simulink model "db5_6_Level_double"  (R2021a)
settings: Solver=VariableStepAuto  StartTime=0.0  StopTime=8  RelTol=1e-3
undefined symbols (not defined in the file): lambda2
libraries: dspsigops x13, dspquant2 x1
(part 2 of 4)

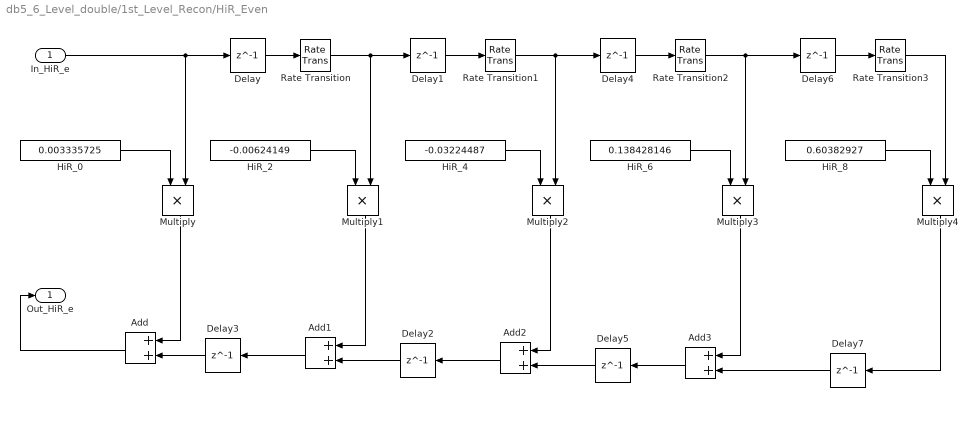
== system db5_6_Level_double/1st_Level_Recon/HiR_Even ==
  In_HiR_e : Inport  OutDataTypeStr=double  SampleTime=1/44100
  Add{,1..3} (4 alike) : Sum  AccumDataTypeStr=double  OutDataTypeStr=double
  Delay{,1..7} (8 alike) : Delay  DelayLength=1  SampleTime=1/44100
  HiR_0 : Constant  Value=0.003335725  OutDataTypeStr=double  SampleTime=1/44100
  HiR_2 : Constant  Value=-0.00624149  OutDataTypeStr=double  SampleTime=1/44100
  HiR_4 : Constant  Value=-0.03224487  OutDataTypeStr=double  SampleTime=1/44100
  HiR_6 : Constant  Value=0.138428146  OutDataTypeStr=double  SampleTime=1/44100
  HiR_8 : Constant  Value=0.60382927  OutDataTypeStr=double  SampleTime=1/44100
  Multiply{,1..4} (5 alike) : Product  OutDataTypeStr=double
  Rate Transition{,1..3} (4 alike) : RateTransition  OutPortSampleTime=1/44100
  Out_HiR_e : Outport  OutDataTypeStr=double  SampleTime=1/44100  VectorParamsAs1DForOutWhenUnconnected=off
  wires:
  Delay3/1 -> Add/2
  In_HiR_e/1 -> Delay/1, Multiply/2
  HiR_4/1 -> Multiply2/1
  Multiply/1 -> Add/1
  Add1/1 -> Delay3/1
  Multiply1/1 -> Add1/1
  Delay2/1 -> Add1/2
  Add/1 -> Out_HiR_e/1
  HiR_0/1 -> Multiply/1
  HiR_2/1 -> Multiply1/1
  Delay1/1 -> Rate Transition1/1
  Rate Transition/1 -> Delay1/1, Multiply1/2
  Rate Transition1/1 -> Delay4/1, Multiply2/2
  Delay/1 -> Rate Transition/1
  Delay4/1 -> Rate Transition2/1
  HiR_6/1 -> Multiply3/1
  Multiply2/1 -> Add2/1
  Add2/1 -> Delay2/1
  Delay5/1 -> Add2/2
  Rate Transition3/1 -> Multiply4/2
  Multiply4/1 -> Delay7/1
  HiR_8/1 -> Multiply4/1
  Rate Transition2/1 -> Delay6/1, Multiply3/2
  Delay6/1 -> Rate Transition3/1
  Add3/1 -> Delay5/1
  Multiply3/1 -> Add3/1
  Delay7/1 -> Add3/2

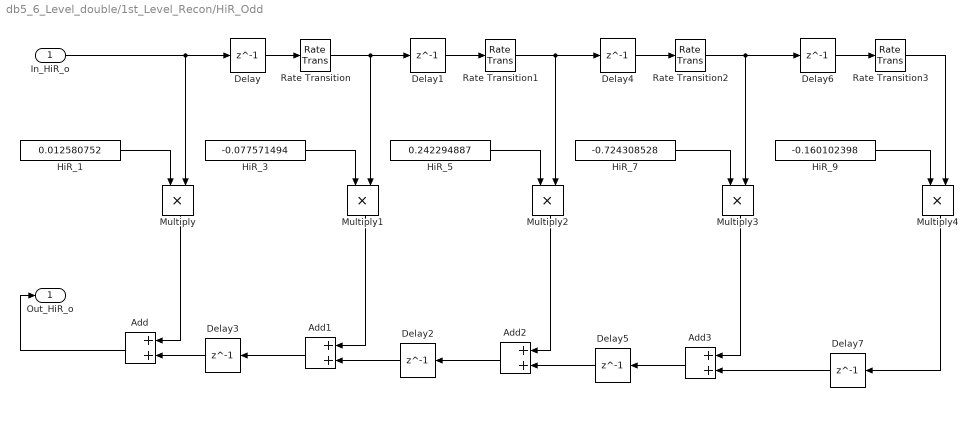
== system db5_6_Level_double/1st_Level_Recon/HiR_Odd ==
  In_HiR_o : Inport  OutDataTypeStr=double  SampleTime=1/44100
  Add{,1..3} (4 alike) : Sum  AccumDataTypeStr=double  OutDataTypeStr=double
  Delay{,1..7} (8 alike) : Delay  DelayLength=1  SampleTime=1/44100
  HiR_1 : Constant  Value=0.012580752  OutDataTypeStr=double  SampleTime=1/44100
  HiR_3 : Constant  Value=-0.077571494  OutDataTypeStr=double  SampleTime=1/44100
  HiR_5 : Constant  Value=0.242294887  OutDataTypeStr=double  SampleTime=1/44100
  HiR_7 : Constant  Value=-0.724308528  OutDataTypeStr=double  SampleTime=1/44100
  HiR_9 : Constant  Value=-0.160102398  OutDataTypeStr=double  SampleTime=1/44100
  Multiply{,1..4} (5 alike) : Product  OutDataTypeStr=double
  Rate Transition{,1..3} (4 alike) : RateTransition  OutPortSampleTime=1/44100
  Out_HiR_o : Outport  OutDataTypeStr=double  SampleTime=1/44100  VectorParamsAs1DForOutWhenUnconnected=off
  wires:
  Add/1 -> Out_HiR_o/1
  Add2/1 -> Delay2/1
  Delay5/1 -> Add2/2
  HiR_9/1 -> Multiply4/1
  HiR_5/1 -> Multiply2/1
  HiR_1/1 -> Multiply/1
  HiR_7/1 -> Multiply3/1
  Multiply1/1 -> Add1/1
  Multiply2/1 -> Add2/1
  Delay2/1 -> Add1/2
  Delay4/1 -> Rate Transition2/1
  Delay3/1 -> Add/2
  In_HiR_o/1 -> Delay/1, Multiply/2
  Rate Transition/1 -> Delay1/1, Multiply1/2
  Rate Transition2/1 -> Delay6/1, Multiply3/2
  Delay7/1 -> Add3/2
  Delay6/1 -> Rate Transition3/1
  Add3/1 -> Delay5/1
  Rate Transition3/1 -> Multiply4/2
  HiR_3/1 -> Multiply1/1
  Multiply3/1 -> Add3/1
  Add1/1 -> Delay3/1
  Multiply4/1 -> Delay7/1
  Multiply/1 -> Add/1
  Rate Transition1/1 -> Delay4/1, Multiply2/2
  Delay1/1 -> Rate Transition1/1
  Delay/1 -> Rate Transition/1

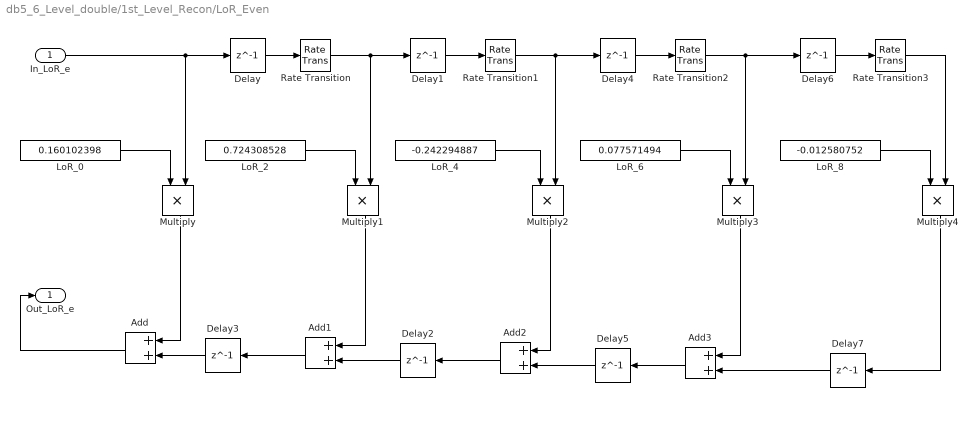
== system db5_6_Level_double/1st_Level_Recon/LoR_Even ==
  In_LoR_e : Inport  OutDataTypeStr=double  SampleTime=1/44100
  Add{,1..3} (4 alike) : Sum  AccumDataTypeStr=double  OutDataTypeStr=double
  Delay{,1..7} (8 alike) : Delay  DelayLength=1  SampleTime=1/44100
  LoR_0 : Constant  Value=0.160102398  OutDataTypeStr=double  SampleTime=1/44100
  LoR_2 : Constant  Value=0.724308528  OutDataTypeStr=double  SampleTime=1/44100
  LoR_4 : Constant  Value=-0.242294887  OutDataTypeStr=double  SampleTime=1/44100
  LoR_6 : Constant  Value=0.077571494  OutDataTypeStr=double  SampleTime=1/44100
  LoR_8 : Constant  Value=-0.012580752  OutDataTypeStr=double  SampleTime=1/44100
  Multiply{,1..4} (5 alike) : Product  OutDataTypeStr=double
  Rate Transition{,1..3} (4 alike) : RateTransition  OutPortSampleTime=1/44100
  Out_LoR_e : Outport  OutDataTypeStr=double  SampleTime=1/44100  VectorParamsAs1DForOutWhenUnconnected=off
  wires:
  Add2/1 -> Delay2/1
  Delay5/1 -> Add2/2
  Add/1 -> Out_LoR_e/1
  Delay1/1 -> Rate Transition1/1
  Rate Transition1/1 -> Delay4/1, Multiply2/2
  Multiply/1 -> Add/1
  Add1/1 -> Delay3/1
  Delay/1 -> Rate Transition/1
  Multiply2/1 -> Add2/1
  Multiply1/1 -> Add1/1
  Delay3/1 -> Add/2
  Delay4/1 -> Rate Transition2/1
  Delay2/1 -> Add1/2
  Rate Transition/1 -> Delay1/1, Multiply1/2
  In_LoR_e/1 -> Delay/1, Multiply/2
  LoR_4/1 -> Multiply2/1
  Delay6/1 -> Rate Transition3/1
  LoR_0/1 -> Multiply/1
  Delay7/1 -> Add3/2
  Rate Transition2/1 -> Delay6/1, Multiply3/2
  LoR_8/1 -> Multiply4/1
  LoR_2/1 -> Multiply1/1
  Rate Transition3/1 -> Multiply4/2
  LoR_6/1 -> Multiply3/1
  Multiply4/1 -> Delay7/1
  Multiply3/1 -> Add3/1
  Add3/1 -> Delay5/1

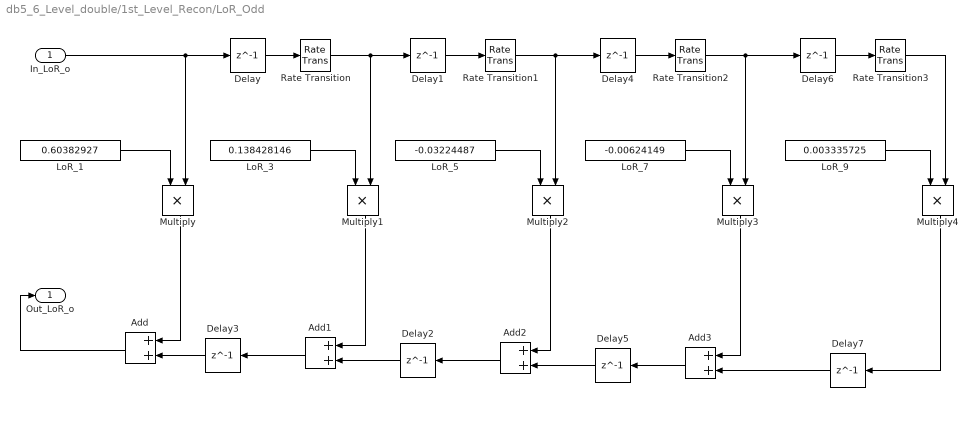
== system db5_6_Level_double/1st_Level_Recon/LoR_Odd ==
  In_LoR_o : Inport  OutDataTypeStr=double  SampleTime=1/44100
  Add{,1..3} (4 alike) : Sum  AccumDataTypeStr=double  OutDataTypeStr=double
  Delay{,1..7} (8 alike) : Delay  DelayLength=1  SampleTime=1/44100
  LoR_1 : Constant  Value=0.60382927  OutDataTypeStr=double  SampleTime=1/44100
  LoR_3 : Constant  Value=0.138428146  OutDataTypeStr=double  SampleTime=1/44100
  LoR_5 : Constant  Value=-0.03224487  OutDataTypeStr=double  SampleTime=1/44100
  LoR_7 : Constant  Value=-0.00624149  OutDataTypeStr=double  SampleTime=1/44100
  LoR_9 : Constant  Value=0.003335725  OutDataTypeStr=double  SampleTime=1/44100
  Multiply{,1..4} (5 alike) : Product  OutDataTypeStr=double
  Rate Transition{,1..3} (4 alike) : RateTransition  OutPortSampleTime=1/44100
  Out_LoR_o : Outport  OutDataTypeStr=double  SampleTime=1/44100  VectorParamsAs1DForOutWhenUnconnected=off
  wires:
  LoR_9/1 -> Multiply4/1
  Rate Transition2/1 -> Delay6/1, Multiply3/2
  Rate Transition/1 -> Delay1/1, Multiply1/2
  Rate Transition3/1 -> Multiply4/2
  Add3/1 -> Delay5/1
  Delay6/1 -> Rate Transition3/1
  Delay7/1 -> Add3/2
  LoR_1/1 -> Multiply/1
  LoR_3/1 -> Multiply1/1
  Delay3/1 -> Add/2
  Delay4/1 -> Rate Transition2/1
  LoR_5/1 -> Multiply2/1
  Delay2/1 -> Add1/2
  Multiply2/1 -> Add2/1
  Add2/1 -> Delay2/1
  LoR_7/1 -> Multiply3/1
  Delay5/1 -> Add2/2
  Multiply3/1 -> Add3/1
  Multiply/1 -> Add/1
  Delay1/1 -> Rate Transition1/1
  Multiply4/1 -> Delay7/1
  In_LoR_o/1 -> Delay/1, Multiply/2
  Add1/1 -> Delay3/1
  Add/1 -> Out_LoR_o/1
  Rate Transition1/1 -> Delay4/1, Multiply2/2
  Delay/1 -> Rate Transition/1
  Multiply1/1 -> Add1/1

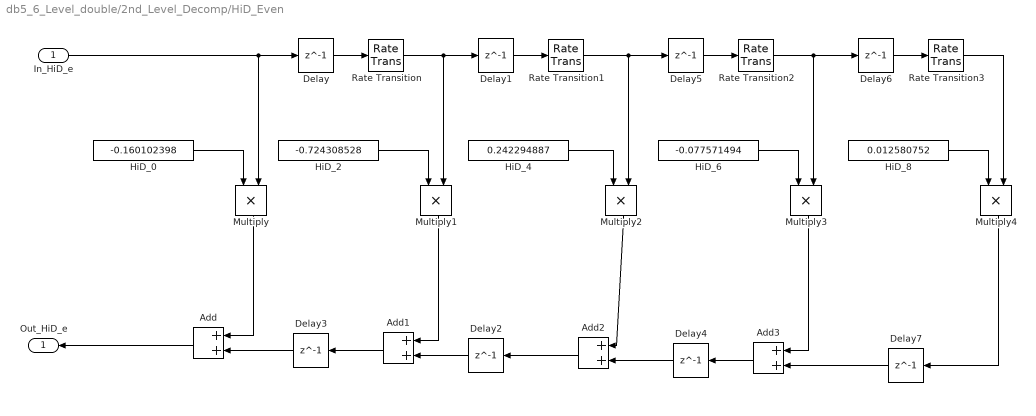
== system db5_6_Level_double/2nd_Level_Decomp/HiD_Even ==
  In_HiD_e : Inport  OutDataTypeStr=double  SampleTime=1/44100
  Add{,1..3} (4 alike) : Sum  AccumDataTypeStr=double  OutDataTypeStr=double
  Delay{,1..7} (8 alike) : Delay  DelayLength=1  SampleTime=1/44100
  HiD_0 : Constant  Value=-0.160102398  OutDataTypeStr=double  SampleTime=1/44100
  HiD_2 : Constant  Value=-0.724308528  OutDataTypeStr=double  SampleTime=1/44100
  HiD_4 : Constant  Value=0.242294887  OutDataTypeStr=double  SampleTime=1/44100
  HiD_6 : Constant  Value=-0.077571494  OutDataTypeStr=double  SampleTime=1/44100
  HiD_8 : Constant  Value=0.012580752  OutDataTypeStr=double  SampleTime=1/44100
  Multiply{,1..4} (5 alike) : Product  OutDataTypeStr=double
  Rate Transition{,1..3} (4 alike) : RateTransition  OutPortSampleTime=1/44100
  Out_HiD_e : Outport  OutDataTypeStr=double  SampleTime=1/44100  VectorParamsAs1DForOutWhenUnconnected=off
  wires:
  Delay1/1 -> Rate Transition1/1
  Delay3/1 -> Add/2
  HiD_2/1 -> Multiply1/1
  Rate Transition2/1 -> Delay6/1, Multiply3/2
  Add/1 -> Out_HiD_e/1
  Delay4/1 -> Add2/2
  Delay5/1 -> Rate Transition2/1
  Rate Transition1/1 -> Delay5/1, Multiply2/2
  HiD_0/1 -> Multiply/1
  Multiply2/1 -> Add2/1
  Add2/1 -> Delay2/1
  HiD_6/1 -> Multiply3/1
  Multiply/1 -> Add/1
  In_HiD_e/1 -> Delay/1, Multiply/2
  Multiply1/1 -> Add1/1
  Rate Transition/1 -> Delay1/1, Multiply1/2
  Add1/1 -> Delay3/1
  HiD_4/1 -> Multiply2/1
  Delay/1 -> Rate Transition/1
  Delay2/1 -> Add1/2
  HiD_8/1 -> Multiply4/1
  Delay6/1 -> Rate Transition3/1
  Rate Transition3/1 -> Multiply4/2
  Multiply4/1 -> Delay7/1
  Multiply3/1 -> Add3/1
  Add3/1 -> Delay4/1
  Delay7/1 -> Add3/2

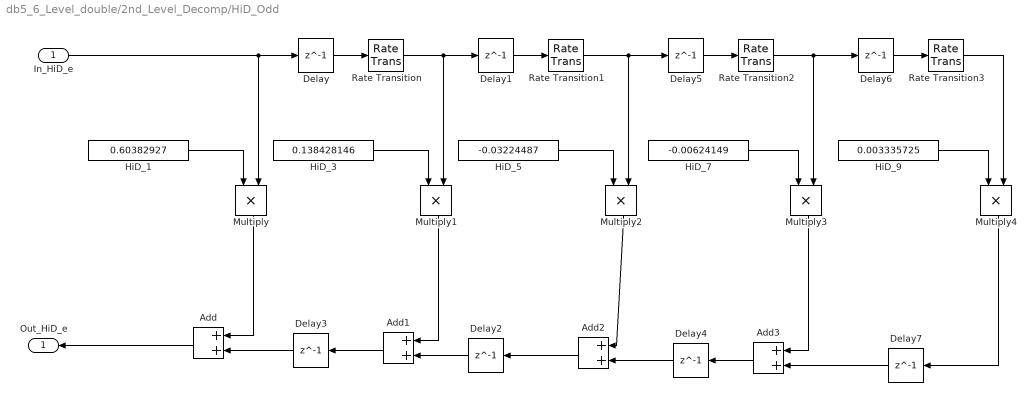
== system db5_6_Level_double/2nd_Level_Decomp/HiD_Odd ==
  In_HiD_e : Inport  OutDataTypeStr=double  SampleTime=1/44100
  Add{,1..3} (4 alike) : Sum  AccumDataTypeStr=double  OutDataTypeStr=double
  Delay{,1..7} (8 alike) : Delay  DelayLength=1  SampleTime=1/44100
  HiD_1 : Constant  Value=0.60382927  OutDataTypeStr=double  SampleTime=1/44100
  HiD_3 : Constant  Value=0.138428146  OutDataTypeStr=double  SampleTime=1/44100
  HiD_5 : Constant  Value=-0.03224487  OutDataTypeStr=double  SampleTime=1/44100
  HiD_7 : Constant  Value=-0.00624149  OutDataTypeStr=double  SampleTime=1/44100
  HiD_9 : Constant  Value=0.003335725  OutDataTypeStr=double  SampleTime=1/44100
  Multiply{,1..4} (5 alike) : Product  OutDataTypeStr=double
  Rate Transition{,1..3} (4 alike) : RateTransition  OutPortSampleTime=1/44100
  Out_HiD_e : Outport  OutDataTypeStr=double  SampleTime=1/44100  VectorParamsAs1DForOutWhenUnconnected=off
  wires:
  Multiply4/1 -> Delay7/1
  Delay6/1 -> Rate Transition3/1
  Rate Transition3/1 -> Multiply4/2
  Add3/1 -> Delay4/1
  Add/1 -> Out_HiD_e/1
  Delay1/1 -> Rate Transition1/1
  Delay7/1 -> Add3/2
  Rate Transition2/1 -> Delay6/1, Multiply3/2
  Delay3/1 -> Add/2
  Rate Transition/1 -> Delay1/1, Multiply1/2
  Rate Transition1/1 -> Delay5/1, Multiply2/2
  Delay4/1 -> Add2/2
  Multiply/1 -> Add/1
  Add2/1 -> Delay2/1
  Delay5/1 -> Rate Transition2/1
  Multiply1/1 -> Add1/1
  Delay2/1 -> Add1/2
  Delay/1 -> Rate Transition/1
  Add1/1 -> Delay3/1
  Multiply3/1 -> Add3/1
  HiD_3/1 -> Multiply1/1
  Multiply2/1 -> Add2/1
  HiD_7/1 -> Multiply3/1
  In_HiD_e/1 -> Delay/1, Multiply/2
  HiD_1/1 -> Multiply/1
  HiD_5/1 -> Multiply2/1
  HiD_9/1 -> Multiply4/1

== system db5_6_Level_double/2nd_Level_Decomp/LoD_Even ==
  In_HiD_e : Inport  OutDataTypeStr=double  SampleTime=1/44100
  Add{,1..3} (4 alike) : Sum  AccumDataTypeStr=double  OutDataTypeStr=double
  Delay{,1..7} (8 alike) : Delay  DelayLength=1  SampleTime=1/44100
  LoD_0 : Constant  Value=0.003335725  OutDataTypeStr=double  SampleTime=1/44100
  LoD_2 : Constant  Value=-0.00624149  OutDataTypeStr=double  SampleTime=1/44100
  LoD_4 : Constant  Value=-0.03224487  OutDataTypeStr=double  SampleTime=1/44100
  LoD_6 : Constant  Value=0.138428146  OutDataTypeStr=double  SampleTime=1/44100
  LoD_8 : Constant  Value=0.60382927  OutDataTypeStr=double  SampleTime=1/44100
  Multiply{,1..4} (5 alike) : Product  OutDataTypeStr=double
  Rate Transition{,1..3} (4 alike) : RateTransition  OutPortSampleTime=1/44100
  Out_HiD_e : Outport  OutDataTypeStr=double  SampleTime=1/44100  VectorParamsAs1DForOutWhenUnconnected=off
  wires:
  Multiply3/1 -> Add3/1
  LoD_4/1 -> Multiply2/1
  Multiply2/1 -> Add2/1
  Add1/1 -> Delay3/1
  Delay2/1 -> Add1/2
  Delay/1 -> Rate Transition/1
  Multiply1/1 -> Add1/1
  In_HiD_e/1 -> Delay/1, Multiply/2
  Add2/1 -> Delay2/1
  Delay5/1 -> Rate Transition2/1
  Multiply/1 -> Add/1
  LoD_8/1 -> Multiply4/1
  Delay4/1 -> Add2/2
  Rate Transition1/1 -> Delay5/1, Multiply2/2
  Rate Transition/1 -> Delay1/1, Multiply1/2
  Delay3/1 -> Add/2
  Rate Transition2/1 -> Delay6/1, Multiply3/2
  Add/1 -> Out_HiD_e/1
  Delay1/1 -> Rate Transition1/1
  Delay7/1 -> Add3/2
  LoD_6/1 -> Multiply3/1
  Add3/1 -> Delay4/1
  Rate Transition3/1 -> Multiply4/2
  Delay6/1 -> Rate Transition3/1
  Multiply4/1 -> Delay7/1
  LoD_2/1 -> Multiply1/1
  LoD_0/1 -> Multiply/1

== system db5_6_Level_double/2nd_Level_Decomp/LoD_Odd ==
  In_HiD_e : Inport  OutDataTypeStr=double  SampleTime=1/44100
  Add{,1..3} (4 alike) : Sum  AccumDataTypeStr=double  OutDataTypeStr=double
  Delay{,1..7} (8 alike) : Delay  DelayLength=1  SampleTime=1/44100
  LoD_1 : Constant  Value=-0.012580752  OutDataTypeStr=double  SampleTime=1/44100
  LoD_3 : Constant  Value=0.077571494  OutDataTypeStr=double  SampleTime=1/44100
  LoD_5 : Constant  Value=-0.242294887  OutDataTypeStr=double  SampleTime=1/44100
  LoD_7 : Constant  Value=0.724308528  OutDataTypeStr=double  SampleTime=1/44100
  LoD_9 : Constant  Value=0.160102398  OutDataTypeStr=double  SampleTime=1/44100
  Multiply{,1..4} (5 alike) : Product  OutDataTypeStr=double
  Rate Transition{,1..3} (4 alike) : RateTransition  OutPortSampleTime=1/44100
  Out_HiD_e : Outport  OutDataTypeStr=double  SampleTime=1/44100  VectorParamsAs1DForOutWhenUnconnected=off
  wires:
  LoD_9/1 -> Multiply4/1
  LoD_3/1 -> Multiply1/1
  LoD_5/1 -> Multiply2/1
  In_HiD_e/1 -> Delay/1, Multiply/2
  LoD_1/1 -> Multiply/1
  Multiply1/1 -> Add1/1
  Multiply3/1 -> Add3/1
  Multiply2/1 -> Add2/1
  Add1/1 -> Delay3/1
  Delay2/1 -> Add1/2
  Delay5/1 -> Rate Transition2/1
  Rate Transition/1 -> Delay1/1, Multiply1/2
  Multiply/1 -> Add/1
  Add2/1 -> Delay2/1
  Delay/1 -> Rate Transition/1
  Delay4/1 -> Add2/2
  Delay3/1 -> Add/2
  Delay7/1 -> Add3/2
  Add/1 -> Out_HiD_e/1
  Delay1/1 -> Rate Transition1/1
  Rate Transition2/1 -> Delay6/1, Multiply3/2
  Rate Transition1/1 -> Delay5/1, Multiply2/2
  LoD_7/1 -> Multiply3/1
  Multiply4/1 -> Delay7/1
  Delay6/1 -> Rate Transition3/1
  Add3/1 -> Delay4/1
  Rate Transition3/1 -> Multiply4/2

== system db5_6_Level_double/2nd_Level_Recon/HiR_Even ==
  In_HiR_e : Inport  OutDataTypeStr=double  SampleTime=1/44100
  Add{,1..3} (4 alike) : Sum  AccumDataTypeStr=double  OutDataTypeStr=double
  Delay{,1..7} (8 alike) : Delay  DelayLength=1  SampleTime=1/44100
  HiR_0 : Constant  Value=0.003335725  OutDataTypeStr=double  SampleTime=1/44100
  HiR_2 : Constant  Value=-0.00624149  OutDataTypeStr=double  SampleTime=1/44100
  HiR_4 : Constant  Value=-0.03224487  OutDataTypeStr=double  SampleTime=1/44100
  HiR_6 : Constant  Value=0.138428146  OutDataTypeStr=double  SampleTime=1/44100
  HiR_8 : Constant  Value=0.60382927  OutDataTypeStr=double  SampleTime=1/44100
  Multiply{,1..4} (5 alike) : Product  OutDataTypeStr=double
  Rate Transition{,1..3} (4 alike) : RateTransition  OutPortSampleTime=1/44100
  Out_HiR_e : Outport  OutDataTypeStr=double  SampleTime=1/44100  VectorParamsAs1DForOutWhenUnconnected=off
  wires:
  Delay3/1 -> Add/2
  In_HiR_e/1 -> Delay/1, Multiply/2
  HiR_4/1 -> Multiply2/1
  Multiply/1 -> Add/1
  Add1/1 -> Delay3/1
  Multiply1/1 -> Add1/1
  Delay2/1 -> Add1/2
  Add/1 -> Out_HiR_e/1
  HiR_0/1 -> Multiply/1
  HiR_2/1 -> Multiply1/1
  Delay1/1 -> Rate Transition1/1
  Rate Transition/1 -> Delay1/1, Multiply1/2
  Rate Transition1/1 -> Delay4/1, Multiply2/2
  Delay/1 -> Rate Transition/1
  Delay4/1 -> Rate Transition2/1
  HiR_6/1 -> Multiply3/1
  Multiply2/1 -> Add2/1
  Add2/1 -> Delay2/1
  Delay5/1 -> Add2/2
  Rate Transition3/1 -> Multiply4/2
  Multiply4/1 -> Delay7/1
  HiR_8/1 -> Multiply4/1
  Rate Transition2/1 -> Delay6/1, Multiply3/2
  Delay6/1 -> Rate Transition3/1
  Add3/1 -> Delay5/1
  Multiply3/1 -> Add3/1
  Delay7/1 -> Add3/2

== system db5_6_Level_double/2nd_Level_Recon/HiR_Odd ==
  In_HiR_o : Inport  OutDataTypeStr=double  SampleTime=1/44100
  Add{,1..3} (4 alike) : Sum  AccumDataTypeStr=double  OutDataTypeStr=double
  Delay{,1..7} (8 alike) : Delay  DelayLength=1  SampleTime=1/44100
  HiR_1 : Constant  Value=0.012580752  OutDataTypeStr=double  SampleTime=1/44100
  HiR_3 : Constant  Value=-0.077571494  OutDataTypeStr=double  SampleTime=1/44100
  HiR_5 : Constant  Value=0.242294887  OutDataTypeStr=double  SampleTime=1/44100
  HiR_7 : Constant  Value=-0.724308528  OutDataTypeStr=double  SampleTime=1/44100
  HiR_9 : Constant  Value=-0.160102398  OutDataTypeStr=double  SampleTime=1/44100
  Multiply{,1..4} (5 alike) : Product  OutDataTypeStr=double
  Rate Transition{,1..3} (4 alike) : RateTransition  OutPortSampleTime=1/44100
  Out_HiR_o : Outport  OutDataTypeStr=double  SampleTime=1/44100  VectorParamsAs1DForOutWhenUnconnected=off
  wires:
  Add/1 -> Out_HiR_o/1
  Add2/1 -> Delay2/1
  Delay5/1 -> Add2/2
  HiR_9/1 -> Multiply4/1
  HiR_5/1 -> Multiply2/1
  HiR_1/1 -> Multiply/1
  HiR_7/1 -> Multiply3/1
  Multiply1/1 -> Add1/1
  Multiply2/1 -> Add2/1
  Delay2/1 -> Add1/2
  Delay4/1 -> Rate Transition2/1
  Delay3/1 -> Add/2
  In_HiR_o/1 -> Delay/1, Multiply/2
  Rate Transition/1 -> Delay1/1, Multiply1/2
  Rate Transition2/1 -> Delay6/1, Multiply3/2
  Delay7/1 -> Add3/2
  Delay6/1 -> Rate Transition3/1
  Add3/1 -> Delay5/1
  Rate Transition3/1 -> Multiply4/2
  HiR_3/1 -> Multiply1/1
  Multiply3/1 -> Add3/1
  Add1/1 -> Delay3/1
  Multiply4/1 -> Delay7/1
  Multiply/1 -> Add/1
  Rate Transition1/1 -> Delay4/1, Multiply2/2
  Delay1/1 -> Rate Transition1/1
  Delay/1 -> Rate Transition/1

== system db5_6_Level_double/2nd_Level_Recon/LoR_Even ==
  In_LoR_e : Inport  OutDataTypeStr=double  SampleTime=1/44100
  Add{,1..3} (4 alike) : Sum  AccumDataTypeStr=double  OutDataTypeStr=double
  Delay{,1..7} (8 alike) : Delay  DelayLength=1  SampleTime=1/44100
  LoR_0 : Constant  Value=0.160102398  OutDataTypeStr=double  SampleTime=1/44100
  LoR_2 : Constant  Value=0.724308528  OutDataTypeStr=double  SampleTime=1/44100
  LoR_4 : Constant  Value=-0.242294887  OutDataTypeStr=double  SampleTime=1/44100
  LoR_6 : Constant  Value=0.077571494  OutDataTypeStr=double  SampleTime=1/44100
  LoR_8 : Constant  Value=-0.012580752  OutDataTypeStr=double  SampleTime=1/44100
  Multiply{,1..4} (5 alike) : Product  OutDataTypeStr=double
  Rate Transition{,1..3} (4 alike) : RateTransition  OutPortSampleTime=1/44100
  Out_LoR_e : Outport  OutDataTypeStr=double  SampleTime=1/44100  VectorParamsAs1DForOutWhenUnconnected=off
  wires:
  Add2/1 -> Delay2/1
  Delay5/1 -> Add2/2
  Add/1 -> Out_LoR_e/1
  Delay1/1 -> Rate Transition1/1
  Rate Transition1/1 -> Delay4/1, Multiply2/2
  Multiply/1 -> Add/1
  Add1/1 -> Delay3/1
  Delay/1 -> Rate Transition/1
  Multiply2/1 -> Add2/1
  Multiply1/1 -> Add1/1
  Delay3/1 -> Add/2
  Delay4/1 -> Rate Transition2/1
  Delay2/1 -> Add1/2
  Rate Transition/1 -> Delay1/1, Multiply1/2
  In_LoR_e/1 -> Delay/1, Multiply/2
  LoR_4/1 -> Multiply2/1
  Delay6/1 -> Rate Transition3/1
  LoR_0/1 -> Multiply/1
  Delay7/1 -> Add3/2
  Rate Transition2/1 -> Delay6/1, Multiply3/2
  LoR_8/1 -> Multiply4/1
  LoR_2/1 -> Multiply1/1
  Rate Transition3/1 -> Multiply4/2
  LoR_6/1 -> Multiply3/1
  Multiply4/1 -> Delay7/1
  Multiply3/1 -> Add3/1
  Add3/1 -> Delay5/1

== system db5_6_Level_double/2nd_Level_Recon/LoR_Odd ==
  In_LoR_o : Inport  OutDataTypeStr=double  SampleTime=1/44100
  Add{,1..3} (4 alike) : Sum  AccumDataTypeStr=double  OutDataTypeStr=double
  Delay{,1..7} (8 alike) : Delay  DelayLength=1  SampleTime=1/44100
  LoR_1 : Constant  Value=0.60382927  OutDataTypeStr=double  SampleTime=1/44100
  LoR_3 : Constant  Value=0.138428146  OutDataTypeStr=double  SampleTime=1/44100
  LoR_5 : Constant  Value=-0.03224487  OutDataTypeStr=double  SampleTime=1/44100
  LoR_7 : Constant  Value=-0.00624149  OutDataTypeStr=double  SampleTime=1/44100
  LoR_9 : Constant  Value=0.003335725  OutDataTypeStr=double  SampleTime=1/44100
  Multiply{,1..4} (5 alike) : Product  OutDataTypeStr=double
  Rate Transition{,1..3} (4 alike) : RateTransition  OutPortSampleTime=1/44100
  Out_LoR_o : Outport  OutDataTypeStr=double  SampleTime=1/44100  VectorParamsAs1DForOutWhenUnconnected=off
  wires:
  LoR_9/1 -> Multiply4/1
  Rate Transition2/1 -> Delay6/1, Multiply3/2
  Rate Transition/1 -> Delay1/1, Multiply1/2
  Rate Transition3/1 -> Multiply4/2
  Add3/1 -> Delay5/1
  Delay6/1 -> Rate Transition3/1
  Delay7/1 -> Add3/2
  LoR_1/1 -> Multiply/1
  LoR_3/1 -> Multiply1/1
  Delay3/1 -> Add/2
  Delay4/1 -> Rate Transition2/1
  LoR_5/1 -> Multiply2/1
  Delay2/1 -> Add1/2
  Multiply2/1 -> Add2/1
  Add2/1 -> Delay2/1
  LoR_7/1 -> Multiply3/1
  Delay5/1 -> Add2/2
  Multiply3/1 -> Add3/1
  Multiply/1 -> Add/1
  Delay1/1 -> Rate Transition1/1
  Multiply4/1 -> Delay7/1
  In_LoR_o/1 -> Delay/1, Multiply/2
  Add1/1 -> Delay3/1
  Add/1 -> Out_LoR_o/1
  Rate Transition1/1 -> Delay4/1, Multiply2/2
  Delay/1 -> Rate Transition/1
  Multiply1/1 -> Add1/1

== system db5_6_Level_double/3rd_Level_Decomp/HiD_Even ==
  In_HiD_e : Inport  OutDataTypeStr=double  SampleTime=1/44100
  Add{,1..3} (4 alike) : Sum  AccumDataTypeStr=double  OutDataTypeStr=double
  Delay{,1..7} (8 alike) : Delay  DelayLength=1  SampleTime=1/44100
  HiD_0 : Constant  Value=-0.160102398  OutDataTypeStr=double  SampleTime=1/44100
  HiD_2 : Constant  Value=-0.724308528  OutDataTypeStr=double  SampleTime=1/44100
  HiD_4 : Constant  Value=0.242294887  OutDataTypeStr=double  SampleTime=1/44100
  HiD_6 : Constant  Value=-0.077571494  OutDataTypeStr=double  SampleTime=1/44100
  HiD_8 : Constant  Value=0.012580752  OutDataTypeStr=double  SampleTime=1/44100
  Multiply{,1..4} (5 alike) : Product  OutDataTypeStr=double
  Rate Transition{,1..3} (4 alike) : RateTransition  OutPortSampleTime=1/44100
  Out_HiD_e : Outport  OutDataTypeStr=double  SampleTime=1/44100  VectorParamsAs1DForOutWhenUnconnected=off
  wires:
  Delay1/1 -> Rate Transition1/1
  Delay3/1 -> Add/2
  HiD_2/1 -> Multiply1/1
  Rate Transition2/1 -> Delay6/1, Multiply3/2
  Add/1 -> Out_HiD_e/1
  Delay4/1 -> Add2/2
  Delay5/1 -> Rate Transition2/1
  Rate Transition1/1 -> Delay5/1, Multiply2/2
  HiD_0/1 -> Multiply/1
  Multiply2/1 -> Add2/1
  Add2/1 -> Delay2/1
  HiD_6/1 -> Multiply3/1
  Multiply/1 -> Add/1
  In_HiD_e/1 -> Delay/1, Multiply/2
  Multiply1/1 -> Add1/1
  Rate Transition/1 -> Delay1/1, Multiply1/2
  Add1/1 -> Delay3/1
  HiD_4/1 -> Multiply2/1
  Delay/1 -> Rate Transition/1
  Delay2/1 -> Add1/2
  HiD_8/1 -> Multiply4/1
  Delay6/1 -> Rate Transition3/1
  Rate Transition3/1 -> Multiply4/2
  Multiply4/1 -> Delay7/1
  Multiply3/1 -> Add3/1
  Add3/1 -> Delay4/1
  Delay7/1 -> Add3/2

== system db5_6_Level_double/3rd_Level_Decomp/HiD_Odd ==
  In_HiD_e : Inport  OutDataTypeStr=double  SampleTime=1/44100
  Add{,1..3} (4 alike) : Sum  AccumDataTypeStr=double  OutDataTypeStr=double
  Delay{,1..7} (8 alike) : Delay  DelayLength=1  SampleTime=1/44100
  HiD_1 : Constant  Value=0.60382927  OutDataTypeStr=double  SampleTime=1/44100
  HiD_3 : Constant  Value=0.138428146  OutDataTypeStr=double  SampleTime=1/44100
  HiD_5 : Constant  Value=-0.03224487  OutDataTypeStr=double  SampleTime=1/44100
  HiD_7 : Constant  Value=-0.00624149  OutDataTypeStr=double  SampleTime=1/44100
  HiD_9 : Constant  Value=0.003335725  OutDataTypeStr=double  SampleTime=1/44100
  Multiply{,1..4} (5 alike) : Product  OutDataTypeStr=double
  Rate Transition{,1..3} (4 alike) : RateTransition  OutPortSampleTime=1/44100
  Out_HiD_e : Outport  OutDataTypeStr=double  SampleTime=1/44100  VectorParamsAs1DForOutWhenUnconnected=off
  wires:
  Multiply4/1 -> Delay7/1
  Delay6/1 -> Rate Transition3/1
  Rate Transition3/1 -> Multiply4/2
  Add3/1 -> Delay4/1
  Add/1 -> Out_HiD_e/1
  Delay1/1 -> Rate Transition1/1
  Delay7/1 -> Add3/2
  Rate Transition2/1 -> Delay6/1, Multiply3/2
  Delay3/1 -> Add/2
  Rate Transition/1 -> Delay1/1, Multiply1/2
  Rate Transition1/1 -> Delay5/1, Multiply2/2
  Delay4/1 -> Add2/2
  Multiply/1 -> Add/1
  Add2/1 -> Delay2/1
  Delay5/1 -> Rate Transition2/1
  Multiply1/1 -> Add1/1
  Delay2/1 -> Add1/2
  Delay/1 -> Rate Transition/1
  Add1/1 -> Delay3/1
  Multiply3/1 -> Add3/1
  HiD_3/1 -> Multiply1/1
  Multiply2/1 -> Add2/1
  HiD_7/1 -> Multiply3/1
  In_HiD_e/1 -> Delay/1, Multiply/2
  HiD_1/1 -> Multiply/1
  HiD_5/1 -> Multiply2/1
  HiD_9/1 -> Multiply4/1

== system db5_6_Level_double/3rd_Level_Decomp/LoD_Even ==
  In_HiD_e : Inport  OutDataTypeStr=double  SampleTime=1/44100
  Add{,1..3} (4 alike) : Sum  AccumDataTypeStr=double  OutDataTypeStr=double
  Delay{,1..7} (8 alike) : Delay  DelayLength=1  SampleTime=1/44100
  LoD_0 : Constant  Value=0.003335725  OutDataTypeStr=double  SampleTime=1/44100
  LoD_2 : Constant  Value=-0.00624149  OutDataTypeStr=double  SampleTime=1/44100
  LoD_4 : Constant  Value=-0.03224487  OutDataTypeStr=double  SampleTime=1/44100
  LoD_6 : Constant  Value=0.138428146  OutDataTypeStr=double  SampleTime=1/44100
  LoD_8 : Constant  Value=0.60382927  OutDataTypeStr=double  SampleTime=1/44100
  Multiply{,1..4} (5 alike) : Product  OutDataTypeStr=double
  Rate Transition{,1..3} (4 alike) : RateTransition  OutPortSampleTime=1/44100
  Out_HiD_e : Outport  OutDataTypeStr=double  SampleTime=1/44100  VectorParamsAs1DForOutWhenUnconnected=off
  wires:
  Multiply3/1 -> Add3/1
  LoD_4/1 -> Multiply2/1
  Multiply2/1 -> Add2/1
  Add1/1 -> Delay3/1
  Delay2/1 -> Add1/2
  Delay/1 -> Rate Transition/1
  Multiply1/1 -> Add1/1
  In_HiD_e/1 -> Delay/1, Multiply/2
  Add2/1 -> Delay2/1
  Delay5/1 -> Rate Transition2/1
  Multiply/1 -> Add/1
  LoD_8/1 -> Multiply4/1
  Delay4/1 -> Add2/2
  Rate Transition1/1 -> Delay5/1, Multiply2/2
  Rate Transition/1 -> Delay1/1, Multiply1/2
  Delay3/1 -> Add/2
  Rate Transition2/1 -> Delay6/1, Multiply3/2
  Add/1 -> Out_HiD_e/1
  Delay1/1 -> Rate Transition1/1
  Delay7/1 -> Add3/2
  LoD_6/1 -> Multiply3/1
  Add3/1 -> Delay4/1
  Rate Transition3/1 -> Multiply4/2
  Delay6/1 -> Rate Transition3/1
  Multiply4/1 -> Delay7/1
  LoD_2/1 -> Multiply1/1
  LoD_0/1 -> Multiply/1

== system db5_6_Level_double/3rd_Level_Decomp/LoD_Odd ==
  In_HiD_e : Inport  OutDataTypeStr=double  SampleTime=1/44100
  Add{,1..3} (4 alike) : Sum  AccumDataTypeStr=double  OutDataTypeStr=double
  Delay{,1..7} (8 alike) : Delay  DelayLength=1  SampleTime=1/44100
  LoD_1 : Constant  Value=-0.012580752  OutDataTypeStr=double  SampleTime=1/44100
  LoD_3 : Constant  Value=0.077571494  OutDataTypeStr=double  SampleTime=1/44100
  LoD_5 : Constant  Value=-0.242294887  OutDataTypeStr=double  SampleTime=1/44100
  LoD_7 : Constant  Value=0.724308528  OutDataTypeStr=double  SampleTime=1/44100
  LoD_9 : Constant  Value=0.160102398  OutDataTypeStr=double  SampleTime=1/44100
  Multiply{,1..4} (5 alike) : Product  OutDataTypeStr=double
  Rate Transition{,1..3} (4 alike) : RateTransition  OutPortSampleTime=1/44100
  Out_HiD_e : Outport  OutDataTypeStr=double  SampleTime=1/44100  VectorParamsAs1DForOutWhenUnconnected=off
  wires:
  LoD_9/1 -> Multiply4/1
  LoD_3/1 -> Multiply1/1
  LoD_5/1 -> Multiply2/1
  In_HiD_e/1 -> Delay/1, Multiply/2
  LoD_1/1 -> Multiply/1
  Multiply1/1 -> Add1/1
  Multiply3/1 -> Add3/1
  Multiply2/1 -> Add2/1
  Add1/1 -> Delay3/1
  Delay2/1 -> Add1/2
  Delay5/1 -> Rate Transition2/1
  Rate Transition/1 -> Delay1/1, Multiply1/2
  Multiply/1 -> Add/1
  Add2/1 -> Delay2/1
  Delay/1 -> Rate Transition/1
  Delay4/1 -> Add2/2
  Delay3/1 -> Add/2
  Delay7/1 -> Add3/2
  Add/1 -> Out_HiD_e/1
  Delay1/1 -> Rate Transition1/1
  Rate Transition2/1 -> Delay6/1, Multiply3/2
  Rate Transition1/1 -> Delay5/1, Multiply2/2
  LoD_7/1 -> Multiply3/1
  Multiply4/1 -> Delay7/1
  Delay6/1 -> Rate Transition3/1
  Add3/1 -> Delay4/1
  Rate Transition3/1 -> Multiply4/2

== system db5_6_Level_double/3rd_Level_Recon/HiR_Even ==
  In_HiR_e : Inport  OutDataTypeStr=double  SampleTime=1/44100
  Add{,1..3} (4 alike) : Sum  AccumDataTypeStr=double  OutDataTypeStr=double
  Delay{,1..7} (8 alike) : Delay  DelayLength=1  SampleTime=1/44100
  HiR_0 : Constant  Value=0.003335725  OutDataTypeStr=double  SampleTime=1/44100
  HiR_2 : Constant  Value=-0.00624149  OutDataTypeStr=double  SampleTime=1/44100
  HiR_4 : Constant  Value=-0.03224487  OutDataTypeStr=double  SampleTime=1/44100
  HiR_6 : Constant  Value=0.138428146  OutDataTypeStr=double  SampleTime=1/44100
  HiR_8 : Constant  Value=0.60382927  OutDataTypeStr=double  SampleTime=1/44100
  Multiply{,1..4} (5 alike) : Product  OutDataTypeStr=double
  Rate Transition{,1..3} (4 alike) : RateTransition  OutPortSampleTime=1/44100
  Out_HiR_e : Outport  OutDataTypeStr=double  SampleTime=1/44100  VectorParamsAs1DForOutWhenUnconnected=off
  wires:
  Delay3/1 -> Add/2
  In_HiR_e/1 -> Delay/1, Multiply/2
  HiR_4/1 -> Multiply2/1
  Multiply/1 -> Add/1
  Add1/1 -> Delay3/1
  Multiply1/1 -> Add1/1
  Delay2/1 -> Add1/2
  Add/1 -> Out_HiR_e/1
  HiR_0/1 -> Multiply/1
  HiR_2/1 -> Multiply1/1
  Delay1/1 -> Rate Transition1/1
  Rate Transition/1 -> Delay1/1, Multiply1/2
  Rate Transition1/1 -> Delay4/1, Multiply2/2
  Delay/1 -> Rate Transition/1
  Delay4/1 -> Rate Transition2/1
  HiR_6/1 -> Multiply3/1
  Multiply2/1 -> Add2/1
  Add2/1 -> Delay2/1
  Delay5/1 -> Add2/2
  Rate Transition3/1 -> Multiply4/2
  Multiply4/1 -> Delay7/1
  HiR_8/1 -> Multiply4/1
  Rate Transition2/1 -> Delay6/1, Multiply3/2
  Delay6/1 -> Rate Transition3/1
  Add3/1 -> Delay5/1
  Multiply3/1 -> Add3/1
  Delay7/1 -> Add3/2

== system db5_6_Level_double/3rd_Level_Recon/HiR_Odd ==
  In_HiR_o : Inport  OutDataTypeStr=double  SampleTime=1/44100
  Add{,1..3} (4 alike) : Sum  AccumDataTypeStr=double  OutDataTypeStr=double
  Delay{,1..7} (8 alike) : Delay  DelayLength=1  SampleTime=1/44100
  HiR_1 : Constant  Value=0.012580752  OutDataTypeStr=double  SampleTime=1/44100
  HiR_3 : Constant  Value=-0.077571494  OutDataTypeStr=double  SampleTime=1/44100
  HiR_5 : Constant  Value=0.242294887  OutDataTypeStr=double  SampleTime=1/44100
  HiR_7 : Constant  Value=-0.724308528  OutDataTypeStr=double  SampleTime=1/44100
  HiR_9 : Constant  Value=-0.160102398  OutDataTypeStr=double  SampleTime=1/44100
  Multiply{,1..4} (5 alike) : Product  OutDataTypeStr=double
  Rate Transition{,1..3} (4 alike) : RateTransition  OutPortSampleTime=1/44100
  Out_HiR_o : Outport  OutDataTypeStr=double  SampleTime=1/44100  VectorParamsAs1DForOutWhenUnconnected=off
  wires:
  Add/1 -> Out_HiR_o/1
  Add2/1 -> Delay2/1
  Delay5/1 -> Add2/2
  HiR_9/1 -> Multiply4/1
  HiR_5/1 -> Multiply2/1
  HiR_1/1 -> Multiply/1
  HiR_7/1 -> Multiply3/1
  Multiply1/1 -> Add1/1
  Multiply2/1 -> Add2/1
  Delay2/1 -> Add1/2
  Delay4/1 -> Rate Transition2/1
  Delay3/1 -> Add/2
  In_HiR_o/1 -> Delay/1, Multiply/2
  Rate Transition/1 -> Delay1/1, Multiply1/2
  Rate Transition2/1 -> Delay6/1, Multiply3/2
  Delay7/1 -> Add3/2
  Delay6/1 -> Rate Transition3/1
  Add3/1 -> Delay5/1
  Rate Transition3/1 -> Multiply4/2
  HiR_3/1 -> Multiply1/1
  Multiply3/1 -> Add3/1
  Add1/1 -> Delay3/1
  Multiply4/1 -> Delay7/1
  Multiply/1 -> Add/1
  Rate Transition1/1 -> Delay4/1, Multiply2/2
  Delay1/1 -> Rate Transition1/1
  Delay/1 -> Rate Transition/1

== system db5_6_Level_double/3rd_Level_Recon/LoR_Even ==
  In_LoR_e : Inport  OutDataTypeStr=double  SampleTime=1/44100
  Add{,1..3} (4 alike) : Sum  AccumDataTypeStr=double  OutDataTypeStr=double
  Delay{,1..7} (8 alike) : Delay  DelayLength=1  SampleTime=1/44100
  LoR_0 : Constant  Value=0.160102398  OutDataTypeStr=double  SampleTime=1/44100
  LoR_2 : Constant  Value=0.724308528  OutDataTypeStr=double  SampleTime=1/44100
  LoR_4 : Constant  Value=-0.242294887  OutDataTypeStr=double  SampleTime=1/44100
  LoR_6 : Constant  Value=0.077571494  OutDataTypeStr=double  SampleTime=1/44100
  LoR_8 : Constant  Value=-0.012580752  OutDataTypeStr=double  SampleTime=1/44100
  Multiply{,1..4} (5 alike) : Product  OutDataTypeStr=double
  Rate Transition{,1..3} (4 alike) : RateTransition  OutPortSampleTime=1/44100
  Out_LoR_e : Outport  OutDataTypeStr=double  SampleTime=1/44100  VectorParamsAs1DForOutWhenUnconnected=off
  wires:
  Add2/1 -> Delay2/1
  Delay5/1 -> Add2/2
  Add/1 -> Out_LoR_e/1
  Delay1/1 -> Rate Transition1/1
  Rate Transition1/1 -> Delay4/1, Multiply2/2
  Multiply/1 -> Add/1
  Add1/1 -> Delay3/1
  Delay/1 -> Rate Transition/1
  Multiply2/1 -> Add2/1
  Multiply1/1 -> Add1/1
  Delay3/1 -> Add/2
  Delay4/1 -> Rate Transition2/1
  Delay2/1 -> Add1/2
  Rate Transition/1 -> Delay1/1, Multiply1/2
  In_LoR_e/1 -> Delay/1, Multiply/2
  LoR_4/1 -> Multiply2/1
  Delay6/1 -> Rate Transition3/1
  LoR_0/1 -> Multiply/1
  Delay7/1 -> Add3/2
  Rate Transition2/1 -> Delay6/1, Multiply3/2
  LoR_8/1 -> Multiply4/1
  LoR_2/1 -> Multiply1/1
  Rate Transition3/1 -> Multiply4/2
  LoR_6/1 -> Multiply3/1
  Multiply4/1 -> Delay7/1
  Multiply3/1 -> Add3/1
  Add3/1 -> Delay5/1

== system db5_6_Level_double/3rd_Level_Recon/LoR_Odd ==
  In_LoR_o : Inport  OutDataTypeStr=double  SampleTime=1/44100
  Add{,1..3} (4 alike) : Sum  AccumDataTypeStr=double  OutDataTypeStr=double
  Delay{,1..7} (8 alike) : Delay  DelayLength=1  SampleTime=1/44100
  LoR_1 : Constant  Value=0.60382927  OutDataTypeStr=double  SampleTime=1/44100
  LoR_3 : Constant  Value=0.138428146  OutDataTypeStr=double  SampleTime=1/44100
  LoR_5 : Constant  Value=-0.03224487  OutDataTypeStr=double  SampleTime=1/44100
  LoR_7 : Constant  Value=-0.00624149  OutDataTypeStr=double  SampleTime=1/44100
  LoR_9 : Constant  Value=0.003335725  OutDataTypeStr=double  SampleTime=1/44100
  Multiply{,1..4} (5 alike) : Product  OutDataTypeStr=double
  Rate Transition{,1..3} (4 alike) : RateTransition  OutPortSampleTime=1/44100
  Out_LoR_o : Outport  OutDataTypeStr=double  SampleTime=1/44100  VectorParamsAs1DForOutWhenUnconnected=off
  wires:
  LoR_9/1 -> Multiply4/1
  Rate Transition2/1 -> Delay6/1, Multiply3/2
  Rate Transition/1 -> Delay1/1, Multiply1/2
  Rate Transition3/1 -> Multiply4/2
  Add3/1 -> Delay5/1
  Delay6/1 -> Rate Transition3/1
  Delay7/1 -> Add3/2
  LoR_1/1 -> Multiply/1
  LoR_3/1 -> Multiply1/1
  Delay3/1 -> Add/2
  Delay4/1 -> Rate Transition2/1
  LoR_5/1 -> Multiply2/1
  Delay2/1 -> Add1/2
  Multiply2/1 -> Add2/1
  Add2/1 -> Delay2/1
  LoR_7/1 -> Multiply3/1
  Delay5/1 -> Add2/2
  Multiply3/1 -> Add3/1
  Multiply/1 -> Add/1
  Delay1/1 -> Rate Transition1/1
  Multiply4/1 -> Delay7/1
  In_LoR_o/1 -> Delay/1, Multiply/2
  Add1/1 -> Delay3/1
  Add/1 -> Out_LoR_o/1
  Rate Transition1/1 -> Delay4/1, Multiply2/2
  Delay/1 -> Rate Transition/1
  Multiply1/1 -> Add1/1

== system db5_6_Level_double/4th_Level_Decomp/HiD_Even ==
  In_HiD_e : Inport  OutDataTypeStr=double  SampleTime=1/44100
  Add{,1..3} (4 alike) : Sum  AccumDataTypeStr=double  OutDataTypeStr=double
  Delay{,1..7} (8 alike) : Delay  DelayLength=1  SampleTime=1/44100
  HiD_0 : Constant  Value=-0.160102398  OutDataTypeStr=double  SampleTime=1/44100
  HiD_2 : Constant  Value=-0.724308528  OutDataTypeStr=double  SampleTime=1/44100
  HiD_4 : Constant  Value=0.242294887  OutDataTypeStr=double  SampleTime=1/44100
  HiD_6 : Constant  Value=-0.077571494  OutDataTypeStr=double  SampleTime=1/44100
  HiD_8 : Constant  Value=0.012580752  OutDataTypeStr=double  SampleTime=1/44100
  Multiply{,1..4} (5 alike) : Product  OutDataTypeStr=double
  Rate Transition{,1..3} (4 alike) : RateTransition  OutPortSampleTime=1/44100
  Out_HiD_e : Outport  OutDataTypeStr=double  SampleTime=1/44100  VectorParamsAs1DForOutWhenUnconnected=off
  wires:
  Delay1/1 -> Rate Transition1/1
  Delay3/1 -> Add/2
  HiD_2/1 -> Multiply1/1
  Rate Transition2/1 -> Delay6/1, Multiply3/2
  Add/1 -> Out_HiD_e/1
  Delay4/1 -> Add2/2
  Delay5/1 -> Rate Transition2/1
  Rate Transition1/1 -> Delay5/1, Multiply2/2
  HiD_0/1 -> Multiply/1
  Multiply2/1 -> Add2/1
  Add2/1 -> Delay2/1
  HiD_6/1 -> Multiply3/1
  Multiply/1 -> Add/1
  In_HiD_e/1 -> Delay/1, Multiply/2
  Multiply1/1 -> Add1/1
  Rate Transition/1 -> Delay1/1, Multiply1/2
  Add1/1 -> Delay3/1
  HiD_4/1 -> Multiply2/1
  Delay/1 -> Rate Transition/1
  Delay2/1 -> Add1/2
  HiD_8/1 -> Multiply4/1
  Delay6/1 -> Rate Transition3/1
  Rate Transition3/1 -> Multiply4/2
  Multiply4/1 -> Delay7/1
  Multiply3/1 -> Add3/1
  Add3/1 -> Delay4/1
  Delay7/1 -> Add3/2

== system db5_6_Level_double/4th_Level_Decomp/HiD_Odd ==
  In_HiD_e : Inport  OutDataTypeStr=double  SampleTime=1/44100
  Add{,1..3} (4 alike) : Sum  AccumDataTypeStr=double  OutDataTypeStr=double
  Delay{,1..7} (8 alike) : Delay  DelayLength=1  SampleTime=1/44100
  HiD_1 : Constant  Value=0.60382927  OutDataTypeStr=double  SampleTime=1/44100
  HiD_3 : Constant  Value=0.138428146  OutDataTypeStr=double  SampleTime=1/44100
  HiD_5 : Constant  Value=-0.03224487  OutDataTypeStr=double  SampleTime=1/44100
  HiD_7 : Constant  Value=-0.00624149  OutDataTypeStr=double  SampleTime=1/44100
  HiD_9 : Constant  Value=0.003335725  OutDataTypeStr=double  SampleTime=1/44100
  Multiply{,1..4} (5 alike) : Product  OutDataTypeStr=double
  Rate Transition{,1..3} (4 alike) : RateTransition  OutPortSampleTime=1/44100
  Out_HiD_e : Outport  OutDataTypeStr=double  SampleTime=1/44100  VectorParamsAs1DForOutWhenUnconnected=off
  wires:
  Multiply4/1 -> Delay7/1
  Delay6/1 -> Rate Transition3/1
  Rate Transition3/1 -> Multiply4/2
  Add3/1 -> Delay4/1
  Add/1 -> Out_HiD_e/1
  Delay1/1 -> Rate Transition1/1
  Delay7/1 -> Add3/2
  Rate Transition2/1 -> Delay6/1, Multiply3/2
  Delay3/1 -> Add/2
  Rate Transition/1 -> Delay1/1, Multiply1/2
  Rate Transition1/1 -> Delay5/1, Multiply2/2
  Delay4/1 -> Add2/2
  Multiply/1 -> Add/1
  Add2/1 -> Delay2/1
  Delay5/1 -> Rate Transition2/1
  Multiply1/1 -> Add1/1
  Delay2/1 -> Add1/2
  Delay/1 -> Rate Transition/1
  Add1/1 -> Delay3/1
  Multiply3/1 -> Add3/1
  HiD_3/1 -> Multiply1/1
  Multiply2/1 -> Add2/1
  HiD_7/1 -> Multiply3/1
  In_HiD_e/1 -> Delay/1, Multiply/2
  HiD_1/1 -> Multiply/1
  HiD_5/1 -> Multiply2/1
  HiD_9/1 -> Multiply4/1

== system db5_6_Level_double/4th_Level_Decomp/LoD_Even ==
  In_HiD_e : Inport  OutDataTypeStr=double  SampleTime=1/44100
  Add{,1..3} (4 alike) : Sum  AccumDataTypeStr=double  OutDataTypeStr=double
  Delay{,1..7} (8 alike) : Delay  DelayLength=1  SampleTime=1/44100
  LoD_0 : Constant  Value=0.003335725  OutDataTypeStr=double  SampleTime=1/44100
  LoD_2 : Constant  Value=-0.00624149  OutDataTypeStr=double  SampleTime=1/44100
  LoD_4 : Constant  Value=-0.03224487  OutDataTypeStr=double  SampleTime=1/44100
  LoD_6 : Constant  Value=0.138428146  OutDataTypeStr=double  SampleTime=1/44100
  LoD_8 : Constant  Value=0.60382927  OutDataTypeStr=double  SampleTime=1/44100
  Multiply{,1..4} (5 alike) : Product  OutDataTypeStr=double
  Rate Transition{,1..3} (4 alike) : RateTransition  OutPortSampleTime=1/44100
  Out_HiD_e : Outport  OutDataTypeStr=double  SampleTime=1/44100  VectorParamsAs1DForOutWhenUnconnected=off
  wires:
  Multiply3/1 -> Add3/1
  LoD_4/1 -> Multiply2/1
  Multiply2/1 -> Add2/1
  Add1/1 -> Delay3/1
  Delay2/1 -> Add1/2
  Delay/1 -> Rate Transition/1
  Multiply1/1 -> Add1/1
  In_HiD_e/1 -> Delay/1, Multiply/2
  Add2/1 -> Delay2/1
  Delay5/1 -> Rate Transition2/1
  Multiply/1 -> Add/1
  LoD_8/1 -> Multiply4/1
  Delay4/1 -> Add2/2
  Rate Transition1/1 -> Delay5/1, Multiply2/2
  Rate Transition/1 -> Delay1/1, Multiply1/2
  Delay3/1 -> Add/2
  Rate Transition2/1 -> Delay6/1, Multiply3/2
  Add/1 -> Out_HiD_e/1
  Delay1/1 -> Rate Transition1/1
  Delay7/1 -> Add3/2
  LoD_6/1 -> Multiply3/1
  Add3/1 -> Delay4/1
  Rate Transition3/1 -> Multiply4/2
  Delay6/1 -> Rate Transition3/1
  Multiply4/1 -> Delay7/1
  LoD_2/1 -> Multiply1/1
  LoD_0/1 -> Multiply/1

== system db5_6_Level_double/4th_Level_Decomp/LoD_Odd ==
  In_HiD_e : Inport  OutDataTypeStr=double  SampleTime=1/44100
  Add{,1..3} (4 alike) : Sum  AccumDataTypeStr=double  OutDataTypeStr=double
  Delay{,1..7} (8 alike) : Delay  DelayLength=1  SampleTime=1/44100
  LoD_1 : Constant  Value=-0.012580752  OutDataTypeStr=double  SampleTime=1/44100
  LoD_3 : Constant  Value=0.077571494  OutDataTypeStr=double  SampleTime=1/44100
  LoD_5 : Constant  Value=-0.242294887  OutDataTypeStr=double  SampleTime=1/44100
  LoD_7 : Constant  Value=0.724308528  OutDataTypeStr=double  SampleTime=1/44100
  LoD_9 : Constant  Value=0.160102398  OutDataTypeStr=double  SampleTime=1/44100
  Multiply{,1..4} (5 alike) : Product  OutDataTypeStr=double
  Rate Transition{,1..3} (4 alike) : RateTransition  OutPortSampleTime=1/44100
  Out_HiD_e : Outport  OutDataTypeStr=double  SampleTime=1/44100  VectorParamsAs1DForOutWhenUnconnected=off
  wires:
  LoD_9/1 -> Multiply4/1
  LoD_3/1 -> Multiply1/1
  LoD_5/1 -> Multiply2/1
  In_HiD_e/1 -> Delay/1, Multiply/2
  LoD_1/1 -> Multiply/1
  Multiply1/1 -> Add1/1
  Multiply3/1 -> Add3/1
  Multiply2/1 -> Add2/1
  Add1/1 -> Delay3/1
  Delay2/1 -> Add1/2
  Delay5/1 -> Rate Transition2/1
  Rate Transition/1 -> Delay1/1, Multiply1/2
  Multiply/1 -> Add/1
  Add2/1 -> Delay2/1
  Delay/1 -> Rate Transition/1
  Delay4/1 -> Add2/2
  Delay3/1 -> Add/2
  Delay7/1 -> Add3/2
  Add/1 -> Out_HiD_e/1
  Delay1/1 -> Rate Transition1/1
  Rate Transition2/1 -> Delay6/1, Multiply3/2
  Rate Transition1/1 -> Delay5/1, Multiply2/2
  LoD_7/1 -> Multiply3/1
  Multiply4/1 -> Delay7/1
  Delay6/1 -> Rate Transition3/1
  Add3/1 -> Delay4/1
  Rate Transition3/1 -> Multiply4/2

== system db5_6_Level_double/4th_Level_Recon/HiR_Even ==
  In_HiR_e : Inport  OutDataTypeStr=double  SampleTime=1/44100
  Add{,1..3} (4 alike) : Sum  AccumDataTypeStr=double  OutDataTypeStr=double
  Delay{,1..7} (8 alike) : Delay  DelayLength=1  SampleTime=1/44100
  HiR_0 : Constant  Value=0.003335725  OutDataTypeStr=double  SampleTime=1/44100
  HiR_2 : Constant  Value=-0.00624149  OutDataTypeStr=double  SampleTime=1/44100
  HiR_4 : Constant  Value=-0.03224487  OutDataTypeStr=double  SampleTime=1/44100
  HiR_6 : Constant  Value=0.138428146  OutDataTypeStr=double  SampleTime=1/44100
  HiR_8 : Constant  Value=0.60382927  OutDataTypeStr=double  SampleTime=1/44100
  Multiply{,1..4} (5 alike) : Product  OutDataTypeStr=double
  Rate Transition{,1..3} (4 alike) : RateTransition  OutPortSampleTime=1/44100
  Out_HiR_e : Outport  OutDataTypeStr=double  SampleTime=1/44100  VectorParamsAs1DForOutWhenUnconnected=off
  wires:
  Delay3/1 -> Add/2
  In_HiR_e/1 -> Delay/1, Multiply/2
  HiR_4/1 -> Multiply2/1
  Multiply/1 -> Add/1
  Add1/1 -> Delay3/1
  Multiply1/1 -> Add1/1
  Delay2/1 -> Add1/2
  Add/1 -> Out_HiR_e/1
  HiR_0/1 -> Multiply/1
  HiR_2/1 -> Multiply1/1
  Delay1/1 -> Rate Transition1/1
  Rate Transition/1 -> Delay1/1, Multiply1/2
  Rate Transition1/1 -> Delay4/1, Multiply2/2
  Delay/1 -> Rate Transition/1
  Delay4/1 -> Rate Transition2/1
  HiR_6/1 -> Multiply3/1
  Multiply2/1 -> Add2/1
  Add2/1 -> Delay2/1
  Delay5/1 -> Add2/2
  Rate Transition3/1 -> Multiply4/2
  Multiply4/1 -> Delay7/1
  HiR_8/1 -> Multiply4/1
  Rate Transition2/1 -> Delay6/1, Multiply3/2
  Delay6/1 -> Rate Transition3/1
  Add3/1 -> Delay5/1
  Multiply3/1 -> Add3/1
  Delay7/1 -> Add3/2

== system db5_6_Level_double/4th_Level_Recon/HiR_Odd ==
  In_HiR_o : Inport  OutDataTypeStr=double  SampleTime=1/44100
  Add{,1..3} (4 alike) : Sum  AccumDataTypeStr=double  OutDataTypeStr=double
  Delay{,1..7} (8 alike) : Delay  DelayLength=1  SampleTime=1/44100
  HiR_1 : Constant  Value=0.012580752  OutDataTypeStr=double  SampleTime=1/44100
  HiR_3 : Constant  Value=-0.077571494  OutDataTypeStr=double  SampleTime=1/44100
  HiR_5 : Constant  Value=0.242294887  OutDataTypeStr=double  SampleTime=1/44100
  HiR_7 : Constant  Value=-0.724308528  OutDataTypeStr=double  SampleTime=1/44100
  HiR_9 : Constant  Value=-0.160102398  OutDataTypeStr=double  SampleTime=1/44100
  Multiply{,1..4} (5 alike) : Product  OutDataTypeStr=double
  Rate Transition{,1..3} (4 alike) : RateTransition  OutPortSampleTime=1/44100
  Out_HiR_o : Outport  OutDataTypeStr=double  SampleTime=1/44100  VectorParamsAs1DForOutWhenUnconnected=off
  wires:
  Add/1 -> Out_HiR_o/1
  Add2/1 -> Delay2/1
  Delay5/1 -> Add2/2
  HiR_9/1 -> Multiply4/1
  HiR_5/1 -> Multiply2/1
  HiR_1/1 -> Multiply/1
  HiR_7/1 -> Multiply3/1
  Multiply1/1 -> Add1/1
  Multiply2/1 -> Add2/1
  Delay2/1 -> Add1/2
  Delay4/1 -> Rate Transition2/1
  Delay3/1 -> Add/2
  In_HiR_o/1 -> Delay/1, Multiply/2
  Rate Transition/1 -> Delay1/1, Multiply1/2
  Rate Transition2/1 -> Delay6/1, Multiply3/2
  Delay7/1 -> Add3/2
  Delay6/1 -> Rate Transition3/1
  Add3/1 -> Delay5/1
  Rate Transition3/1 -> Multiply4/2
  HiR_3/1 -> Multiply1/1
  Multiply3/1 -> Add3/1
  Add1/1 -> Delay3/1
  Multiply4/1 -> Delay7/1
  Multiply/1 -> Add/1
  Rate Transition1/1 -> Delay4/1, Multiply2/2
  Delay1/1 -> Rate Transition1/1
  Delay/1 -> Rate Transition/1

== system db5_6_Level_double/4th_Level_Recon/LoR_Even ==
  In_LoR_e : Inport  OutDataTypeStr=double  SampleTime=1/44100
  Add{,1..3} (4 alike) : Sum  AccumDataTypeStr=double  OutDataTypeStr=double
  Delay{,1..7} (8 alike) : Delay  DelayLength=1  SampleTime=1/44100
  LoR_0 : Constant  Value=0.160102398  OutDataTypeStr=double  SampleTime=1/44100
  LoR_2 : Constant  Value=0.724308528  OutDataTypeStr=double  SampleTime=1/44100
  LoR_4 : Constant  Value=-0.242294887  OutDataTypeStr=double  SampleTime=1/44100
  LoR_6 : Constant  Value=0.077571494  OutDataTypeStr=double  SampleTime=1/44100
  LoR_8 : Constant  Value=-0.012580752  OutDataTypeStr=double  SampleTime=1/44100
  Multiply{,1..4} (5 alike) : Product  OutDataTypeStr=double
  Rate Transition{,1..3} (4 alike) : RateTransition  OutPortSampleTime=1/44100
  Out_LoR_e : Outport  OutDataTypeStr=double  SampleTime=1/44100  VectorParamsAs1DForOutWhenUnconnected=off
  wires:
  Add2/1 -> Delay2/1
  Delay5/1 -> Add2/2
  Add/1 -> Out_LoR_e/1
  Delay1/1 -> Rate Transition1/1
  Rate Transition1/1 -> Delay4/1, Multiply2/2
  Multiply/1 -> Add/1
  Add1/1 -> Delay3/1
  Delay/1 -> Rate Transition/1
  Multiply2/1 -> Add2/1
  Multiply1/1 -> Add1/1
  Delay3/1 -> Add/2
  Delay4/1 -> Rate Transition2/1
  Delay2/1 -> Add1/2
  Rate Transition/1 -> Delay1/1, Multiply1/2
  In_LoR_e/1 -> Delay/1, Multiply/2
  LoR_4/1 -> Multiply2/1
  Delay6/1 -> Rate Transition3/1
  LoR_0/1 -> Multiply/1
  Delay7/1 -> Add3/2
  Rate Transition2/1 -> Delay6/1, Multiply3/2
  LoR_8/1 -> Multiply4/1
  LoR_2/1 -> Multiply1/1
  Rate Transition3/1 -> Multiply4/2
  LoR_6/1 -> Multiply3/1
  Multiply4/1 -> Delay7/1
  Multiply3/1 -> Add3/1
  Add3/1 -> Delay5/1

== system db5_6_Level_double/4th_Level_Recon/LoR_Odd ==
  In_LoR_o : Inport  OutDataTypeStr=double  SampleTime=1/44100
  Add{,1..3} (4 alike) : Sum  AccumDataTypeStr=double  OutDataTypeStr=double
  Delay{,1..7} (8 alike) : Delay  DelayLength=1  SampleTime=1/44100
  LoR_1 : Constant  Value=0.60382927  OutDataTypeStr=double  SampleTime=1/44100
  LoR_3 : Constant  Value=0.138428146  OutDataTypeStr=double  SampleTime=1/44100
  LoR_5 : Constant  Value=-0.03224487  OutDataTypeStr=double  SampleTime=1/44100
  LoR_7 : Constant  Value=-0.00624149  OutDataTypeStr=double  SampleTime=1/44100
  LoR_9 : Constant  Value=0.003335725  OutDataTypeStr=double  SampleTime=1/44100
  Multiply{,1..4} (5 alike) : Product  OutDataTypeStr=double
  Rate Transition{,1..3} (4 alike) : RateTransition  OutPortSampleTime=1/44100
  Out_LoR_o : Outport  OutDataTypeStr=double  SampleTime=1/44100  VectorParamsAs1DForOutWhenUnconnected=off
  wires:
  LoR_9/1 -> Multiply4/1
  Rate Transition2/1 -> Delay6/1, Multiply3/2
  Rate Transition/1 -> Delay1/1, Multiply1/2
  Rate Transition3/1 -> Multiply4/2
  Add3/1 -> Delay5/1
  Delay6/1 -> Rate Transition3/1
  Delay7/1 -> Add3/2
  LoR_1/1 -> Multiply/1
  LoR_3/1 -> Multiply1/1
  Delay3/1 -> Add/2
  Delay4/1 -> Rate Transition2/1
  LoR_5/1 -> Multiply2/1
  Delay2/1 -> Add1/2
  Multiply2/1 -> Add2/1
  Add2/1 -> Delay2/1
  LoR_7/1 -> Multiply3/1
  Delay5/1 -> Add2/2
  Multiply3/1 -> Add3/1
  Multiply/1 -> Add/1
  Delay1/1 -> Rate Transition1/1
  Multiply4/1 -> Delay7/1
  In_LoR_o/1 -> Delay/1, Multiply/2
  Add1/1 -> Delay3/1
  Add/1 -> Out_LoR_o/1
  Rate Transition1/1 -> Delay4/1, Multiply2/2
  Delay/1 -> Rate Transition/1
  Multiply1/1 -> Add1/1

== system db5_6_Level_double/5th_Level_Decomp/HiD_Even ==
  In_HiD_e : Inport  OutDataTypeStr=double  SampleTime=1/44100
  Add{,1..3} (4 alike) : Sum  AccumDataTypeStr=double  OutDataTypeStr=double
  Delay{,1..7} (8 alike) : Delay  DelayLength=1  SampleTime=1/44100
  HiD_0 : Constant  Value=-0.160102398  OutDataTypeStr=double  SampleTime=1/44100
  HiD_2 : Constant  Value=-0.724308528  OutDataTypeStr=double  SampleTime=1/44100
  HiD_4 : Constant  Value=0.242294887  OutDataTypeStr=double  SampleTime=1/44100
  HiD_6 : Constant  Value=-0.077571494  OutDataTypeStr=double  SampleTime=1/44100
  HiD_8 : Constant  Value=0.012580752  OutDataTypeStr=double  SampleTime=1/44100
  Multiply{,1..4} (5 alike) : Product  OutDataTypeStr=double
  Rate Transition{,1..3} (4 alike) : RateTransition  OutPortSampleTime=1/44100
  Out_HiD_e : Outport  OutDataTypeStr=double  SampleTime=1/44100  VectorParamsAs1DForOutWhenUnconnected=off
  wires:
  Delay1/1 -> Rate Transition1/1
  Delay3/1 -> Add/2
  HiD_2/1 -> Multiply1/1
  Rate Transition2/1 -> Delay6/1, Multiply3/2
  Add/1 -> Out_HiD_e/1
  Delay4/1 -> Add2/2
  Delay5/1 -> Rate Transition2/1
  Rate Transition1/1 -> Delay5/1, Multiply2/2
  HiD_0/1 -> Multiply/1
  Multiply2/1 -> Add2/1
  Add2/1 -> Delay2/1
  HiD_6/1 -> Multiply3/1
  Multiply/1 -> Add/1
  In_HiD_e/1 -> Delay/1, Multiply/2
  Multiply1/1 -> Add1/1
  Rate Transition/1 -> Delay1/1, Multiply1/2
  Add1/1 -> Delay3/1
  HiD_4/1 -> Multiply2/1
  Delay/1 -> Rate Transition/1
  Delay2/1 -> Add1/2
  HiD_8/1 -> Multiply4/1
  Delay6/1 -> Rate Transition3/1
  Rate Transition3/1 -> Multiply4/2
  Multiply4/1 -> Delay7/1
  Multiply3/1 -> Add3/1
  Add3/1 -> Delay4/1
  Delay7/1 -> Add3/2
